simulink model "feedbackcontrol_II_HW3"  (R2015b)
settings: Solver=VariableStepAuto  StartTime=0.0  StopTime=20  RelTol=1e-3
settings Model: Creator=言厚  LastModifiedBy=言厚

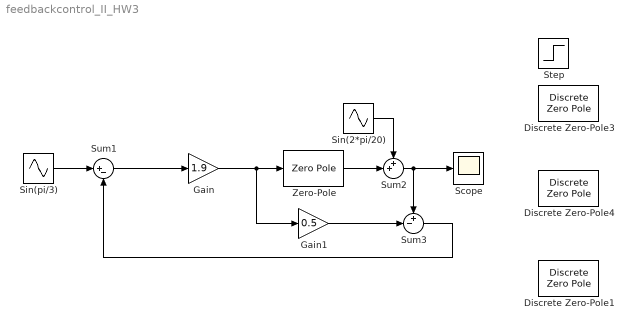
== system feedbackcontrol_II_HW3 ==
  Discrete Zero-Pole1 : DiscreteZeroPole  Zeros=[-0.5]  Poles=[1.4 0.9]  Gain=1
  Discrete Zero-Pole3 : DiscreteZeroPole  Zeros=[0 -0.5]  Poles=[1.4 0.9]  Gain=0.9
  Discrete Zero-Pole4 : DiscreteZeroPole  Zeros=[1.4 0.9]  Poles=[0 -0.5]  Gain=1
  Gain : Gain  Gain=1.9
  Gain1 : Gain  Gain=0.5
  Scope : Scope
  Sin(2*pi/20) : Sin  Amplitude=0.2  Frequency=2*pi/20  SampleTime=0
  Sin(pi/3) : Sin  Frequency=pi/3  SampleTime=0
  Step : Step  Time=0  SampleTime=0
  Sum1 : Sum  Inputs=|+-
  Sum2 : Sum  Inputs=++|
  Sum3 : Sum  Inputs=+-|
  Zero-Pole : ZeroPole  Zeros=[-0.5]  Poles=[1.4 0.9]
  wires:
  Sin(pi/3)/1 -> Sum1/1
  Sum2/1 -> Scope/1, Sum3/1
  Sum1/1 -> Gain/1
  Sum3/1 -> Sum1/2
  Gain1/1 -> Sum3/2
  Zero-Pole/1 -> Sum2/2
  Gain/1 -> Gain1/1, Zero-Pole/1
  Sin(2*pi/20)/1 -> Sum2/1
